simulink model "robot"  (Simulink 6.4)
settings: Solver=FixedStepDiscrete  StartTime=0.0  StopTime=5  FixedStep=0.01  RelTol=1e-3
libraries: RT x1
settings Model: LastModifiedBy=jborges
settings RTWCC: SystemTargetFile=rtwin.tlc  TemplateMakefile=rtwin.tmf  Description=Real-Time Windows Target  ProcessScript=rtwin_make_rtw_hook
settings RTWinTargetCC: TargetFcnLib=ansi_tfl_tmw.mat  GenFloatMathFcnCalls=ANSI_C  ModelReferenceCompliant=off  IncludeERTFirstTime=on  CCOptimize=on

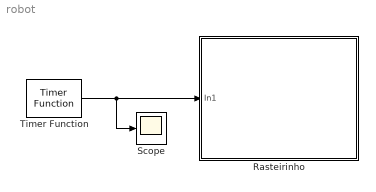
== system robot ==
  Rasteirinho : Subsystem
      mask Display: image(imread('Rasteirinho.bmp'))
  Scope : Scope
      settings: TimeRange=3  YMin=0  YMax=100
  Timer Function : RT/Timer Function  Priority=285810440  step=10  priority=HIGH  ThPriority=TIME CRITICAL
  wires:
  Timer Function/1 -> Rasteirinho/1(In1), Scope/1

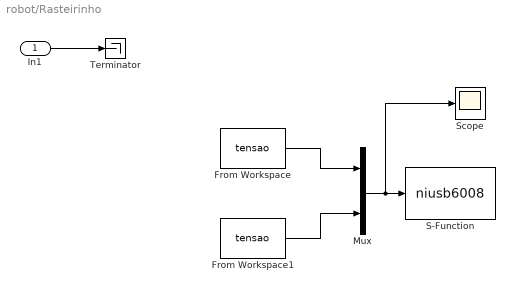
== system robot/Rasteirinho ==
  In1 : Inport
  From Workspace : FromWorkspace  VariableName=tensao  SampleTime=0.01
  From Workspace1 : FromWorkspace  VariableName=tensao  SampleTime=0.01
  Mux : Mux  Inputs=2
  S-Function : S-Function  FunctionName=niusb6008
  Scope : Scope
  Terminator : Terminator
  wires:
  In1/1 -> Terminator/1
  Mux/1 -> S-Function/1, Scope/1
  From Workspace/1 -> Mux/1
  From Workspace1/1 -> Mux/2
